simulink model "AKF_CT1"  (Simulink 6.6)
settings: Solver=ode45  StartTime=0.0  StopTime=1.99  RelTol=1e-3
undefined symbols (not defined in the file): DiscIntNeverNeededParam
libraries: dspstat3 x2, commseqgen2 x2, commutil2 x2, dspbuff3 x1
settings Model: Creator=Home  LastModifiedBy=Мама Люда  SimulationMode=accelerator
settings OptimizationCC: InlineInvariantSignals=on
settings DebuggingCC: SignalResolutionControl=TryResolveAllWithWarning  MultiTaskDSMMsg=warning  MultiTaskCondExecSysMsg=none  StrictBusMsg=None
settings RTWCC: IncludeERTFirstTime=on

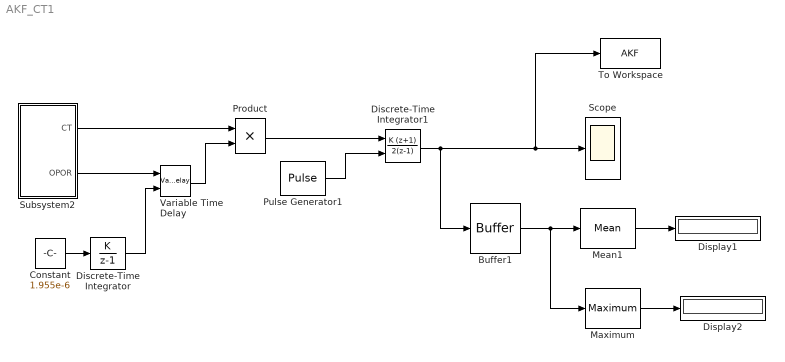
== system AKF_CT1 ==
  Buffer1 : dspbuff3/Buffer  N=1022  V=0  ic=0
  Constant : Constant  Value=1.955e-6  SampleTime=1e-3
  Discrete-Time Integrator : DiscreteIntegrator  IntegratorMethod=Accumulation: Forward Euler  gainval=1  SampleTime=1e-3  ICPrevOutput=DiscIntNeverNeededParam  ICPrevScaledInput=DiscIntNeverNeededParam
  Discrete-Time Integrator1 : DiscreteIntegrator  IntegratorMethod=Accumulation: Trapezoidal  gainval=1/511  ExternalReset=falling  SampleTime=1.955e-6  ICPrevOutput=DiscIntNeverNeededParam  ICPrevScaledInput=DiscIntNeverNeededParam
  Display1 : Display
  Display2 : Display
  Maximum : dspstat3/Maximum  DialogController=dspfixptddg.MinMax  DialogControllerArgs=DataTag0  fcn=Value  reset=None  indexBase=One  operateOver=Each column  colComp=on  operation=maximum  roundingMode=Floor  overflowMode=off
  Mean1 : dspstat3/Mean  DialogController=dspDDGCreate  DialogControllerArgs=DataTag1  run=off  reset_popup=None  roundingMode=Floor  overflowMode=off
  Product : Product  RndMeth=Zero
  Pulse Generator1 : DiscretePulseGenerator  PulseType=Time based  Period=1e-3  PulseWidth=50  PhaseDelay=0.5e-3
  Scope : Scope
      settings: TimeRange=1  YMin=-1  YMax=1  SampleInput=on  SampleTime=1e-3
  Subsystem2 : Subsystem
  To Workspace : ToWorkspace  VariableName=AKF  SampleTime=1e-3  SaveFormat=Array
  Variable Time Delay : VariableTransportDelay  MaximumDelay=1024
  wires:
  Subsystem2/1(CT) -> Product/1
  Product/1 -> Discrete-Time Integrator1/1
  Pulse Generator1/1 -> Discrete-Time Integrator1/2
  Subsystem2/2(OPOR) -> Variable Time Delay/1
  Variable Time Delay/1 -> Product/2
  Discrete-Time Integrator/1 -> Variable Time Delay/2
  Constant/1 -> Discrete-Time Integrator/1
  Discrete-Time Integrator1/1 -> Buffer1/1, Scope/1, To Workspace/1
  Mean1/1 -> Display1/1
  Buffer1/1 -> Mean1/1, Maximum/1
  Maximum/1 -> Display2/1

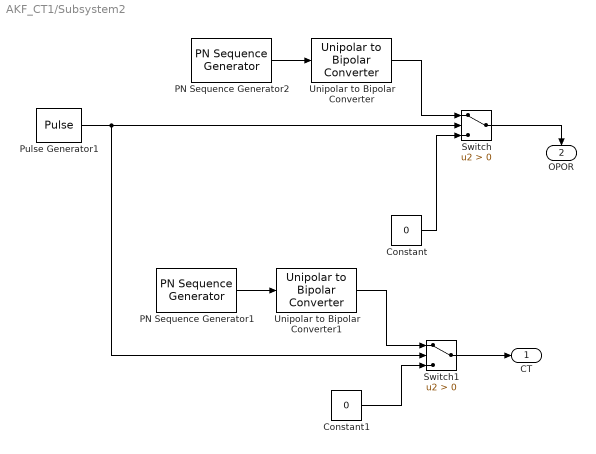
== system AKF_CT1/Subsystem2 ==
  Constant : Constant  Value=0
  Constant1 : Constant  Value=0
  PN Sequence Generator1 : commseqgen2/PN Sequence Generator  poly=[9 4 0]  ini_sta=[1 0 1 1 0 1 1 1 1]  outBitMaskSource=Dialog parameter  shift=0  Ts=1.955e-6  frameBased=off  sampPerFrame=1  reset=off  bitPackedOutputs=off  outDataType=boolean  numPackedBits=8  bitPackDataSigned=off  bitPackedOutDType=double
  PN Sequence Generator2 : commseqgen2/PN Sequence Generator  poly=[9 5 0]  ini_sta=[1 1 1 1 1 1 1 1 1]  outBitMaskSource=Dialog parameter  shift=0  Ts=1.955e-6  frameBased=off  sampPerFrame=1  reset=off  bitPackedOutputs=off  outDataType=boolean  numPackedBits=8  bitPackDataSigned=off  bitPackedOutDType=double
  Pulse Generator1 : DiscretePulseGenerator  PulseType=Time based  Period=2e-3  PulseWidth=50
  Switch : Switch  Criteria=u2 > Threshold
  Switch1 : Switch  Criteria=u2 > Threshold
  Unipolar to Bipolar Converter : commutil2/Unipolar to Bipolar Converter  SystemSampleTime=-1  M=2  polarity=Positive  dataType=double
  Unipolar to Bipolar Converter1 : commutil2/Unipolar to Bipolar Converter  SystemSampleTime=-1  M=2  polarity=Positive  dataType=double
  CT : Outport
  OPOR : Outport  Orientation=down  Port=2
  wires:
  PN Sequence Generator2/1 -> Unipolar to Bipolar Converter/1
  Unipolar to Bipolar Converter/1 -> Switch/1
  Pulse Generator1/1 -> Switch/2, Switch1/2
  Switch/1 -> OPOR/1
  Constant/1 -> Switch/3
  PN Sequence Generator1/1 -> Unipolar to Bipolar Converter1/1
  Unipolar to Bipolar Converter1/1 -> Switch1/1
  Constant1/1 -> Switch1/3
  Switch1/1 -> CT/1
